simulink model "fm"  (R2013a)
settings: Solver=ode45  StartTime=0  StopTime=20e-3  MaxStep=0.01e-3  RelTol=1e-3
settings Model: Creator=B407  LastModifiedBy=B407

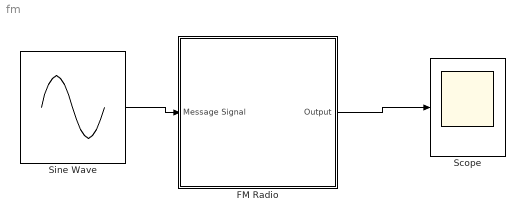
== system fm ==
  "FM Radio " : Subsystem  mask(FM Signal){fm=100, fc=1000, b=5}
      mask prompts: fm "Enter message freq"; fc "enter carrier freq"; b "Enter modulation index"
      mask help: Fm Signal
      mask Help: Fm Signal help
      mask Display: image('b747.jpg')
  Scope : Scope
      settings: TimeRange=0.02  YMin=-1  YMax=1
  Sine Wave : Sin  Frequency=2*pi*100  Phase=pi/2  SampleTime=0
  wires:
  "FM Radio "/1("Output ") -> Scope/1
  Sine Wave/1 -> "FM Radio "/1("Message Signal ")

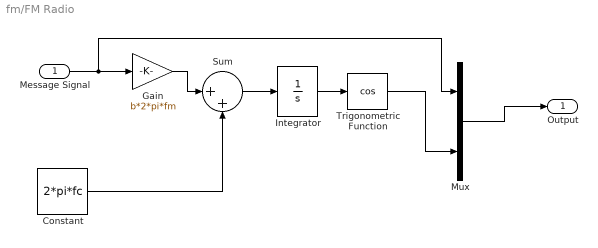
== system fm/FM Radio  ==
  "Message Signal " : Inport
  Constant : Constant  Value=2*pi*fc
  Gain : Gain  Gain=b*2*pi*fm
  Integrator : Integrator
  Mux : Mux  Inputs=2
  Sum : Sum  Inputs=|++
  Trigonometric Function : Trigonometry  Operator=cos
  "Output " : Outport
  wires:
  Gain/1 -> Sum/1
  Sum/1 -> Integrator/1
  Integrator/1 -> Trigonometric Function/1
  "Message Signal "/1 -> Mux/1, Gain/1
  Trigonometric Function/1 -> Mux/2
  Mux/1 -> "Output "/1
  Constant/1 -> Sum/2
